simulink model "LinearMPC_constraints"  (R2021b)
settings: Solver=FixedStepDiscrete  StartTime=0.0  StopTime=tsim  FixedStep=Ts  RelTol=1e-3  EnableMultiTasking=on
values from neighbouring files (symbols this model uses):
  A = sysd.A    [es_4.m]
  B = sysd.B    [es_4.m]
  C_states = eye(2)    [es_4.m]
  D_states = [0 0]'    [es_4.m]
  N = 5    [es_4.m]
  Q_LQsat = Q_LQ/1000    [es_4.m]
  QMPC = Q_LQ    [es_4.m]
  R = R_LQ    (= 1)    [es_4.m]
  sat_max = umax    (= 5)    [es_4.m]
  sat_min = umin    (= -5)    [es_4.m]
  sysd = c2d(sys,Ts)    [es_4.m]
  Ts = 0.1    [es_4.m]
  umax = 5    [es_4.m]
  umin = -5    [es_4.m]
  x0 = [0 10]'    [es_4.m]
  xref = [0 0]'    [es_4.m]
undefined symbols (not defined in the file or in its folder): mympc, Pr, Pr_LQsat
settings Model: Creator=Mirko  LastModifiedBy=Chiara
settings SolverCC: AlgebraicLoopSolver=TrustRegion
settings DataIOCC: LimitDataPoints=on  SaveFormat=Array  SignalLoggingSaveFormat=ModelDataLogs  ReturnWorkspaceOutputs=off
settings OptimizationCC: ExpressionDepthLimit=2147483647  LifeSpan=inf
settings DebuggingCC: UnderspecifiedInitializationDetection=Classic  MergeDetectMultiDrivingBlocksExec=none  SolverPrmCheckMsg=warning  FcnCallInpInsideContextMsg=warning  StateNameClashWarn=warning  SFUnexpectedBacktrackingDiag=warning  SFNoUnconditionalDefaultTransitionDiag=warning  SFExecutionAtInitializationDiag=none  SFMachineParentedDataDiag=warning  ArithmeticOperatorsInVariantConditions=warning
settings HardwareCC: ProdBitPerPointer=32  ProdBitPerSizeT=32  ProdBitPerPtrDiffT=32  ProdLargestAtomicFloat=None  ProdIntDivRoundTo=Undefined  ProdEndianess=Unspecified  ProdWordSize=32  ProdHWDeviceType=32-bit Generic
settings ModelReferenceCC: PropagateSignalLabelsOutOfModel=off
settings SFSimCC: SimUseLocalCustomCode=off  CustomCodeUndefinedFunction=UseInterfaceOnly
settings RTWCC: RTWUseLocalCustomCode=off
settings CodeAppCC: StateflowObjectComments=on
settings GRTTargetCC: TargetLangStandard=C89/C90 (ANSI)
settings ConfigComp: CovMetricSettings=dw  CovSaveCumulativeToWorkspaceVar=on  CovSaveSingleToWorkspaceVar=on  CovExternalEMLEnable=off  CovSFcnEnable=off

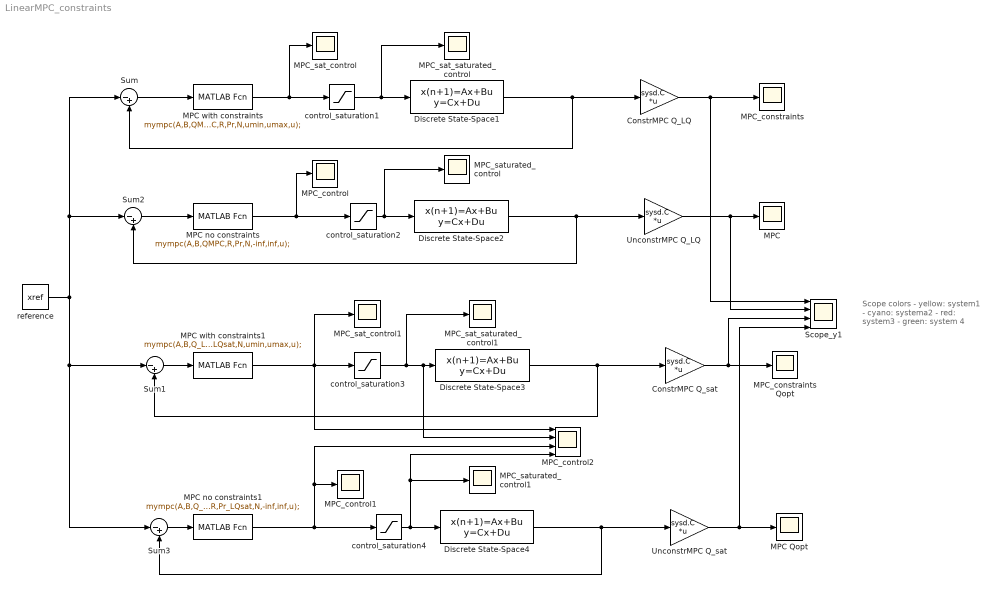
== system LinearMPC_constraints ==
  note: Scope colors
      | - yellow: system1
      | - cyano: systema2
      | - red: system3
      | - green: system 4
  ConstrMPC Q_LQ : Gain  Gain=sysd.C  Multiplication=Matrix(K*u) (u vector)
  ConstrMPC Q_sat : Gain  Gain=sysd.C  Multiplication=Matrix(K*u) (u vector)
  Discrete State-Space{1..4} (4 alike) : DiscreteStateSpace  A=sysd.A  B=sysd.B  C=C_states  D=D_states  InitialCondition=x0  SampleTime=Ts
  MPC : Scope
  MPC Qopt : Scope
  MPC no constraints : MATLABFcn  MATLABFcn=mympc(A,B,QMPC,R,Pr,N,-inf,inf,u);  OutputDimensions=1
  MPC no constraints1 : MATLABFcn  MATLABFcn=mympc(A,B,Q_LQsat,R,Pr_LQsat,N,-inf,inf,u);  OutputDimensions=1
  MPC with constraints : MATLABFcn  MATLABFcn=mympc(A,B,QMPC,R,Pr,N,umin,umax,u);  OutputDimensions=1
  MPC with constraints1 : MATLABFcn  MATLABFcn=mympc(A,B,Q_LQsat,R,Pr_LQsat,N,umin,umax,u);  OutputDimensions=1
  MPC_constraints : Scope
  MPC_constraints Qopt : Scope
  MPC_control : Scope
  MPC_control1 : Scope
  MPC_control2 : Scope  NumInputPorts=4
  MPC_sat_control : Scope
  MPC_sat_control1 : Scope
  MPC_sat_saturated_control : Scope
  MPC_sat_saturated_control1 : Scope
  MPC_saturated_control : Scope
  MPC_saturated_control1 : Scope
  Scope_y1 : Scope  NumInputPorts=4
  Sum{,1..3} (4 alike) : Sum  Inputs=|-+
  UnconstrMPC Q_LQ : Gain  Gain=sysd.C  Multiplication=Matrix(K*u) (u vector)
  UnconstrMPC Q_sat : Gain  Gain=sysd.C  Multiplication=Matrix(K*u) (u vector)
  control_saturation{1..4} (4 alike) : Saturate  UpperLimit=sat_max  LowerLimit=sat_min
  reference : Constant  Value=xref
  wires:
  Discrete State-Space1/1 -> ConstrMPC Q_LQ/1, Sum/2
  Sum/1 -> MPC with constraints/1
  MPC with constraints/1 -> control_saturation1/1, MPC_sat_control/1
  ConstrMPC Q_LQ/1 -> MPC_constraints/1, Scope_y1/1
  control_saturation1/1 -> Discrete State-Space1/1, MPC_sat_saturated_control/1
  Discrete State-Space2/1 -> UnconstrMPC Q_LQ/1, Sum2/2
  MPC no constraints/1 -> control_saturation2/1, MPC_control/1
  UnconstrMPC Q_LQ/1 -> Scope_y1/2, MPC/1
  control_saturation2/1 -> MPC_saturated_control/1, Discrete State-Space2/1
  Sum2/1 -> MPC no constraints/1
  Sum3/1 -> MPC no constraints1/1
  Discrete State-Space4/1 -> UnconstrMPC Q_sat/1, Sum3/2
  control_saturation4/1 -> MPC_control2/4, MPC_saturated_control1/1, Discrete State-Space4/1
  UnconstrMPC Q_sat/1 -> MPC Qopt/1, Scope_y1/4
  MPC no constraints1/1 -> control_saturation4/1, MPC_control2/3, MPC_control1/1
  ConstrMPC Q_sat/1 -> Scope_y1/3, MPC_constraints Qopt/1
  Discrete State-Space3/1 -> ConstrMPC Q_sat/1, Sum1/2
  control_saturation3/1 -> MPC_control2/2, Discrete State-Space3/1, MPC_sat_saturated_control1/1
  MPC with constraints1/1 -> MPC_control2/1, control_saturation3/1, MPC_sat_control1/1
  Sum1/1 -> MPC with constraints1/1
  reference/1 -> Sum1/1, Sum3/1, Sum/1, Sum2/1
